simulink model "Dualactiveconverter_seminar"  (R2024a)
settings: Solver=VariableStepAuto  StartTime=0.0  StopTime=5  RelTol=1e-3
undefined symbols (not defined in the file): C_LV, RC_LV
libraries: spsIGBTDiodeLib x8, spsSeriesRLCBranchLib x2, spsDCVoltageSourceLib x2, spsVoltageMeasurementLib x2, spsLinearTransformerLib x1, simulink x1, spsSawtoothGeneratorLib x1, spspowerguiLib x1
settings Model: Creator=farza  LastModifiedBy=farza

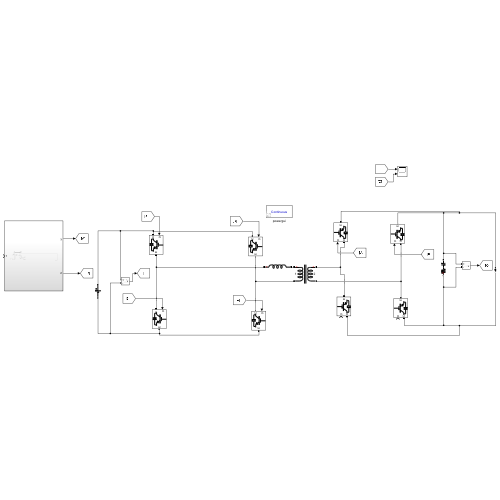
[thumbnail: Simulink's stored preview of the top-level diagram]
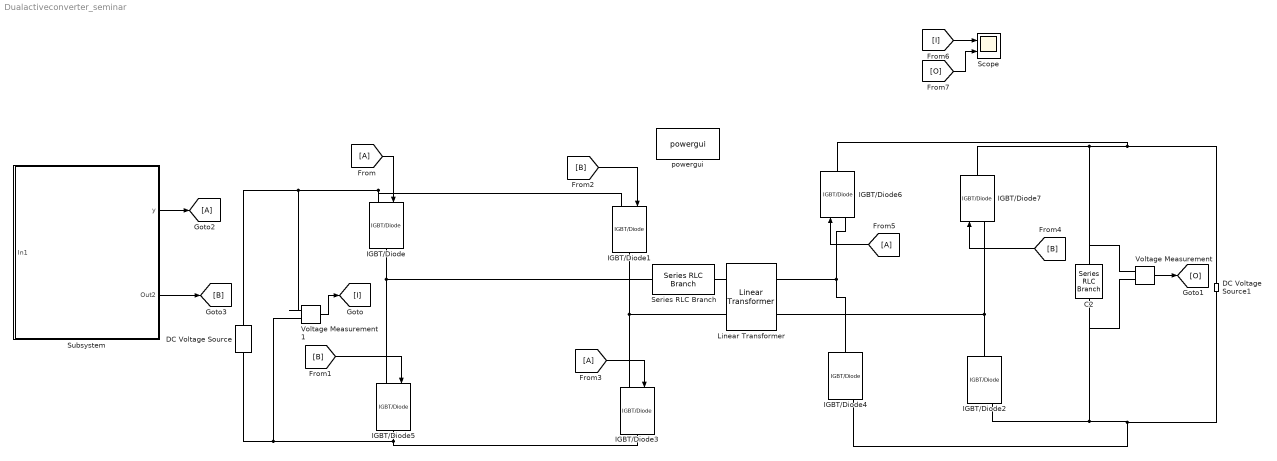
== system Dualactiveconverter_seminar ==
  C2 : spsSeriesRLCBranchLib/Series RLC Branch  LConnTagsString=__new0  RConnTagsString=__new0  BranchType=RC  Resistance=RC_LV  Inductance=1  SetiL0=off  InitialCurrent=0  Capacitance=C_LV  Setx0=off  InitialVoltage=0  Measurements=None
  DC Voltage Source : spsDCVoltageSourceLib/DC Voltage Source  Amplitude=300  Measurements=None
  DC Voltage Source1 : spsDCVoltageSourceLib/DC Voltage Source  Amplitude=30  Measurements=None
  From : From
  From3 : From
  From5 : From
  Goto2 : Goto
  IGBT/Diode{,1..7} (8 alike) : spsIGBTDiodeLib/IGBT//Diode  Ron=1e-3  Rs=1e5  Cs=inf  Measurements=off
  Linear Transformer : spsLinearTransformerLib/Linear Transformer  UNITS=SI  NominalPower=[ 250e6 60 ]  winding1=[7.35e+05 4.3218 0.45856]  winding2=[3.15e+05 0.7938 0.084225]  ThreeWindings=off  winding3=[3.15e+05 0.7938 0.084225]  RmLm=[1.0804e+06 2866]  Measurements=None  DataType=on
  Scope : Scope  NumInputPorts=2
  Series RLC Branch : spsSeriesRLCBranchLib/Series RLC Branch  LConnTagsString=__new0  RConnTagsString=__new0  BranchType=L  Resistance=1  Inductance=1.5e-05  SetiL0=off  InitialCurrent=0  Capacitance=1e-6  Setx0=off  InitialVoltage=0  Measurements=None
  Subsystem : Subsystem
  Voltage Measurement : spsVoltageMeasurementLib/Voltage Measurement  PhasorSimulation=off  OutputType=Complex  PSBequivalent=0
  Voltage Measurement1 : spsVoltageMeasurementLib/Voltage Measurement  PhasorSimulation=off  OutputType=Complex  PSBequivalent=0
  powergui : spspowerguiLib/powergui  Priority=1  SimulationMode=Continuous  SampleTime=50e-6  frequency=60  Iterations=50  frequencyindice=0  Pbase=100e6  ErrMax=1e-4  UnitsV=kV  UnitsW=MW  buscounter=0  FunctionMessages=off  echomessages=off  EnableUseOfTLC=off  CurrentSourceSwitches=off  DisableSnubberDevices=off  DisableRonSwitches=off  DisableVfSwitches=off  DisplayEquations=off  AutomaticDiscreteSolvers=off  SolverType=Tustin/Backward Euler (TBE)  Interpol=off  ExternalGateDelay=off  methode=off  Ts=100  x0status=blocks  SPID=on  SwTol=0  HookPort=off  NonlinearTolerance=0  nMaxIteration=15  ContinueOnMaxIteration=off  RestoreLinks=warning  ResistiveCurrentMeasurement=off  Frange=[0:2:500]  Ylog=off  Xlog=on  ShowGrid=off  save=off  variable=ZData  structure=0  ZoomFFT=off  StartTime=0.0  cycles=1  DisplayStyle=1  fundamental=60  FreqAxis=off  MaxFrequency=1000  frequencyindicesteady=1  RmsSteady=1  display=off
  wires:
  [B] -> IGBT/Diode5/1
  [B] -> IGBT/Diode1/1
  From3/1 -> IGBT/Diode3/1
  From/1 -> IGBT/Diode/1
  Subsystem/1(y) -> Goto2/1
  Subsystem/2(Out2) -> [B]
  From5/1 -> IGBT/Diode6/1
  [B] -> IGBT/Diode7/1
  Voltage Measurement1/1 -> [I]
  [O] -> Scope/2
  [I] -> Scope/1
  Voltage Measurement/1 -> [O]
  connections:
  IGBT/Diode5/LConn1 -- Series RLC Branch/LConn1 -- IGBT/Diode/RConn1
  IGBT/Diode1/RConn1 -- Linear Transformer/LConn2 -- IGBT/Diode3/LConn1
  DC Voltage Source/LConn1 -- Voltage Measurement1/LConn2 -- IGBT/Diode5/RConn1 -- IGBT/Diode3/RConn1
  DC Voltage Source/RConn1 -- Voltage Measurement1/LConn1 -- IGBT/Diode/LConn1 -- IGBT/Diode1/LConn1
  Linear Transformer/LConn1 -- Series RLC Branch/RConn1
  IGBT/Diode6/RConn1 -- DC Voltage Source1/RConn1 -- Voltage Measurement/LConn1 -- C2/RConn1 -- IGBT/Diode7/RConn1
  IGBT/Diode7/LConn1 -- Linear Transformer/RConn2 -- IGBT/Diode2/RConn1
  IGBT/Diode4/RConn1 -- Linear Transformer/RConn1 -- IGBT/Diode6/LConn1
  IGBT/Diode4/LConn1 -- DC Voltage Source1/LConn1 -- Voltage Measurement/LConn2 -- C2/LConn1 -- IGBT/Diode2/LConn1

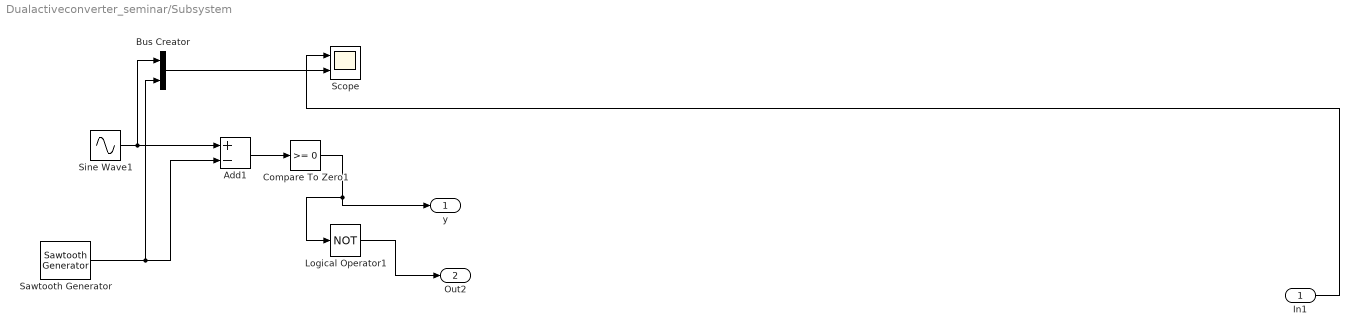
== system Dualactiveconverter_seminar/Subsystem ==
  In1 : Inport
  Add1 : Sum  Inputs=+-
  Bus Creator : BusCreator  Inputs=2
  Compare To Zero1 : simulink/Logic and Bit Operations/Compare To Zero  relop=>=  OutDataTypeStr=boolean
  Logical Operator1 : Logic  Operator=NOT  AllPortsSameDT=off  OutDataTypeStr=boolean
  Sawtooth Generator : spsSawtoothGeneratorLib/Sawtooth Generator  Freq=1000  Phase=0  Ts=0
  Scope : Scope  NumInputPorts=2
  Sine Wave1 : Sin  Frequency=2*pi*50  Phase=pi  SampleTime=0
  y : Outport
  Out2 : Outport  Port=2
  wires:
  In1/1 -> Scope/1
  Sine Wave1/1 -> Bus Creator/1, Add1/1
  Sawtooth Generator/1 -> Bus Creator/2, Add1/2
  Logical Operator1/1 -> Out2/1
  Add1/1 -> Compare To Zero1/1
  Compare To Zero1/1 -> y/1, Logical Operator1/1
  Bus Creator/1 -> Scope/2
